simulink library "AEMS_Standard_Library"  (R2016b)
settings: Solver=ode45  StartTime=0.0  StopTime=10.0  RelTol=1e-3
undefined symbols (not defined in the file or in its folder): BkPY, carto, Cbx_extegr, Cbx_lpegrsys, Cbx_portegr, Cnx_bnk_nr_conf, Cnx_cyl_nr_conf, ConfigManagement, configuration_management, Cxx_dcm_io_tmr_end_xxxx, Cxx_dcm_rt_tmr_end, Cxx_DID_xxxx_IO_max, Cxx_DID_xxxx_IO_min, Cxx_egrhsofs, Cxx_vmaniegi, DEM_DEBOUNCE_FREEZE, DEM_DTR_CTL_INVISIBLE, DEM_DTR_CTL_NORMAL, Dem_DtrId2_XXX, Dem_DtrId3_XXX, Dem_DtrId4_XXX, Dem_DtrId5_XXX, Dem_DtrId6_XXX, Dem_DtrId7_XXX, Dem_DtrId8_XXX, Dem_DtrId9_XXX, Dem_DtrId_XXX, Dem_EnableConditionId2_XXX, Dem_EnableConditionId3_XXX, Dem_EnableConditionId4_XXX, Dem_EnableConditionId5_XXX, Dem_EnableConditionId6_XXX, Dem_EnableConditionId7_XXX, Dem_EnableConditionId8_XXX, Dem_EnableConditionId_XXX, Dem_EventId, Dem_EventId2_XXX, Dem_EventId3_XXX, Dem_EventId4_XXX, Dem_EventId5_XXX, Dem_EventId6_XXX, Dem_EventId7_XXX, Dem_EventId8_XXX, Dem_EventId9_XXX, Dem_EventId_Device_Faulttype, Dem_EventId_XXX, DEM_IUMPR_GENERAL_DENOMINATOR, DEM_OPCYC_IGNITION, Dem_RatioId2_XXX, Dem_RatioId3_XXX, Dem_RatioId4_XXX, Dem_RatioId5_XXX, Dem_RatioId6_XXX, Dem_RatioId7_XXX, Dem_RatioId8_XXX, Dem_RatioId_XXX, Dem_StorageConditionId2_XXX, Dem_StorageConditionId3_XXX, Dem_StorageConditionId4_XXX, Dem_StorageConditionId5_XXX ... (+65)
libraries: AEMS_Standard_Library x477, simulink x2
(part 26 of 39)

== system AEMS_Standard_Library/COM/AEMS_FRAME_SUPERVISION/ecu_frm_detection ==
  Clear_Diag_Info : Inport
  Frm_Detection_Cnd : Inport  Port=2
  Frm_Conf : Inport  Port=3
  Status_Loc2 : Inport  Port=4
  AEMS_NVM_SET : AEMS_Standard_Library/MEM/AEMS_NVM_SET  Tag=[LIB]  initial_value=0
      settings: AttributesFormatString=<initial=%<initial_value>>
  C_mngt : Subsystem
      settings: RTWSystemCode=Nonreusable function
  Frame_Detected : Outport
  wires:
  AEMS_NVM_SET/1 -> C_mngt/5(Frm_Detected_PREV)
  C_mngt/1(Frm_Detected) -> AEMS_NVM_SET/1, Frame_Detected/1
  Frm_Detection_Cnd/1 -> C_mngt/1(Frm_Detection_Cnd)
  Frm_Conf/1 -> C_mngt/3(Frm_Conf)
  Status_Loc2/1 -> C_mngt/2(Status_Loc2)
  Clear_Diag_Info/1 -> C_mngt/4(Clear_Diag_Info_Counter)

== system AEMS_Standard_Library/COM/AEMS_FRAME_SUPERVISION/ecu_frm_monitoring ==
  rcpt_frm : Inport
  JT1 : Inport  Port=2
  JT2 : Inport  Port=3
  TimeSched_dt : Inport  Port=4
  GADE : Inport  Port=5
  ECU_Category : Inport  Port=6
  IgnitionSupplyConfirmation : Inport  Port=7
  Specific_Mon_Cnd : Inport  Port=8
  Frame_Detected : Inport  Port=9
  BCM_Status : Inport  Port=10
  USM_Status : Inport  Port=11
  Vbx_atsr_sys_ecu_ini_task10ms : Inport  Port=12
  A_Monitoring_Condition : Subsystem
      settings: RTWSystemCode=Nonreusable function
  B_Status_Management : Subsystem
  Status : Outport
      settings: AttributesFormatString=%<SignalName>
  Mon_Authorize : Outport  Port=2
  wires:
  Vbx_atsr_sys_ecu_ini_task10ms/1 -> B_Status_Management/6(Vbx_atsr_sys_ecu_ini_task10ms)
  rcpt_frm/1 -> B_Status_Management/1(rcpt_frm)
  TimeSched_dt/1 -> B_Status_Management/3(TimeSched_dt)
  JT1/1 -> B_Status_Management/4(JT1)
  JT2/1 -> B_Status_Management/5(JT2)
  Frame_Detected/1 -> A_Monitoring_Condition/5(Frame_Detected_Loc2), B_Status_Management/7(Frame_Detected)
  ECU_Category/1 -> A_Monitoring_Condition/2(ECU_Category)
  Specific_Mon_Cnd/1 -> A_Monitoring_Condition/4(Specific_Mon_Cnd)
  USM_Status/1 -> A_Monitoring_Condition/7(USM_Status)
  IgnitionSupplyConfirmation/1 -> A_Monitoring_Condition/3(IgnitionSupplyConfirmation)
  GADE/1 -> A_Monitoring_Condition/1(GADE)
  BCM_Status/1 -> A_Monitoring_Condition/6(BCM_Status)
  A_Monitoring_Condition/1(Mon_Authorize) -> B_Status_Management/2(Mon_Authorize), Mon_Authorize/1
  B_Status_Management/1(Status) -> Status/1

== system AEMS_Standard_Library/COM/AEMS_FRAME_SUPERVISION/ecu_monitoring_display ==
  rcpt_frm_dspl : Inport
  ClearDiagInfo_dspl : Inport  Port=2
  IGN_Status : Inport  Port=3
  Dspl_Mask_Cnd : Inport  Port=4
  Status : Inport  Port=5
  M_Absent_ini : Inport  Port=6
  decM : Inport  Port=7
  decThres : Inport  Port=8
  VALMAX : Inport  Port=9
  Mon_Authorized : Inport  Port=10
  Vbx_atsr_sys_ecu_ini_task10ms : Inport  Port=11
  Constant2 : Constant  Value=0  OutDataTypeStr=Inherit: Inherit via back propagation
  Constant3 : Constant  Value=false
  D_ctr_mem_max : Subsystem
  E_diag_display : Subsystem
  Switch : Switch  Criteria=u2 ~= 0
      settings: AttributesFormatString=Criteria=%<Criteria>
  Switch1 : Switch  Criteria=u2 ~= 0
      settings: AttributesFormatString=Criteria=%<Criteria>
  Switch2 : Switch  Criteria=u2 ~= 0
      settings: AttributesFormatString=Criteria=%<Criteria>
  Unit Delay : UnitDelay  SampleTime=-1
      settings: AttributesFormatString=<initial=%<InitialCondition>>
  Unit Delay1 : UnitDelay  SampleTime=-1
      settings: AttributesFormatString=<initial=%<InitialCondition>>
  Diagnosis_Byte : Outport
  M_Absent : Outport  Port=2
  wires:
  Unit Delay1/1 -> D_ctr_mem_max/2(M_Absent_PREV)
  Unit Delay/1 -> D_ctr_mem_max/3(Vbx_rcpt_XXX_mon_PREV)
  Switch/1 -> M_Absent/1, E_diag_display/1(M_Absent), Unit Delay1/1
  Switch1/1 -> Unit Delay/1
  ClearDiagInfo_dspl/1 -> D_ctr_mem_max/8(Clear_Diag_Info_Counter)
  rcpt_frm_dspl/1 -> D_ctr_mem_max/7(Frame_Received_Counter)
  Vbx_atsr_sys_ecu_ini_task10ms/1 -> Switch1/2, Switch/2, Switch2/2
  Constant2/1 -> Switch2/1
  E_diag_display/1(Diagnosis_Byte) -> Switch2/3
  Constant3/1 -> Switch1/1
  D_ctr_mem_max/2(Vbx_rcpt_XXX_mon) -> Switch1/3
  M_Absent_ini/1 -> Switch/1
  D_ctr_mem_max/1(M_Absent) -> Switch/3
  Switch2/1 -> Diagnosis_Byte/1
  VALMAX/1 -> D_ctr_mem_max/1(VALMAX)
  Dspl_Mask_Cnd/1 -> E_diag_display/3(Dspl_Mask_Cnd)
  Status/1 -> D_ctr_mem_max/9(Status), E_diag_display/4(Status)
  Mon_Authorized/1 -> E_diag_display/2(Mon_Authorized)
  decM/1 -> D_ctr_mem_max/5(decM)
  decThres/1 -> D_ctr_mem_max/6(decThres)
  IGN_Status/1 -> D_ctr_mem_max/4(IGN_Status)

== system AEMS_Standard_Library/DCM/AEMS_APP_REQUEST_IOCONTROL/Request_IOControl_Subsystem ==
  Req_stadj_xxxx : Inport
  Req_rcecu_xxxx : Inport  Port=2
  Generic_Condition : Inport  Port=3
  Specific_Condition_xxxx : Inport  Port=4
  Req_tmr_end_xxxx : Inport  Port=5
  AEMS_EDGE_RISING : AEMS_Standard_Library/EDGE/AEMS_EDGE_RISING  Tag=[LIB]  init=true
      settings: AttributesFormatString=|
      | %<MaskType>
      | Initial Value : %<init>
  AEMS_SRFLIPFLOP : AEMS_Standard_Library/FLAG/AEMS_SRFLIPFLOP  Tag=[LIB]  init=false
      settings: AttributesFormatString=%<MaskType>\nInitial condition (state of Q): = %<init>
  Logical Operator : Logic  Operator=OR  Inputs=3  OutDataTypeStr=boolean
  Logical Operator1 : Logic  OutDataTypeStr=boolean
  Logical Operator2 : Logic  Operator=NOT  OutDataTypeStr=boolean
  Logical_Operator1 : Logic  Operator=XOR  OutDataTypeStr=boolean
  Logical_Operator4 : Logic  Operator=XOR  OutDataTypeStr=boolean
  Unit Delay : UnitDelay  InitialCondition=false  SampleTime=-1
      settings: AttributesFormatString=<initial=%<InitialCondition>>
  Unit Delay1 : UnitDelay  InitialCondition=false  SampleTime=-1
      settings: AttributesFormatString=<initial=%<InitialCondition>>
  Flag_io_request_xxxx : Outport
  Flag_dcm_io_tmr_end_xxxx : Outport  Port=2
  wires:
  Req_stadj_xxxx/1 -> Logical_Operator4/1, Unit Delay/1
  Unit Delay/1 -> Logical_Operator4/2
  Logical_Operator4/1 -> AEMS_SRFLIPFLOP/1
  Req_rcecu_xxxx/1 -> Logical_Operator1/1, Unit Delay1/1
  Generic_Condition/1 -> Logical Operator1/1
  Specific_Condition_xxxx/1 -> Logical Operator1/2
  Unit Delay1/1 -> Logical_Operator1/2
  Logical_Operator1/1 -> Logical Operator/1
  Logical Operator/1 -> AEMS_SRFLIPFLOP/2
  Logical Operator1/1 -> Logical Operator2/1
  Logical Operator2/1 -> Logical Operator/2
  AEMS_SRFLIPFLOP/1 -> Flag_io_request_xxxx/1
  Req_tmr_end_xxxx/1 -> AEMS_EDGE_RISING/1
  AEMS_EDGE_RISING/1 -> Logical Operator/3, Flag_dcm_io_tmr_end_xxxx/1

== system AEMS_Standard_Library/DCM/AEMS_APP_REQUEST_IOCONTROL/Timer_IOControl_Subsystem ==
  note: Reset Threshold value defined in
      | Cxx_dcm_io_tmr_end_xxxx whenever
      | a edge raising or failing detected
  note: Decrementation:
      | Decrement 10 milisecondes from Calibration High_Threshold to 0 and set the Duration of Timer
      | Decrement every 10MS
  note: Set Timer value
      | Set Timer_End if Duration reached
  Req_stadj_xxxx : Inport
  Constant : Constant  Value=0  OutDataTypeStr=single
  Cxx_dcm_io_tmr_end_xxxx : Constant  Value=Cxx_dcm_io_tmr_end_xxxx  OutDataTypeStr=single
  Increment : Constant  Value=10  OutDataTypeStr=single
  Logical_Operator4 : Logic  Operator=XOR  OutDataTypeStr=boolean
  MinMax : MinMax  Function=max  Inputs=2
  Relational Operator : RelationalOperator  Operator=<=  OutDataTypeStr=boolean  RndMeth=Nearest  InputSameDT=on
  Saturation : Saturate  UpperLimit=655350  LowerLimit=0
      settings: AttributesFormatString=<limits=%<UpperLimit>/%<LowerLimit>>
  Sum : Sum  Inputs=-+  OutDataTypeStr=single  SaturateOnIntegerOverflow=on  InputSameDT=on
      settings: AttributesFormatString=SAT = %<SaturateOnIntegerOverflow>
  Switch : Switch  Criteria=u2 ~= 0
      settings: AttributesFormatString=Criteria=%<Criteria>
  Unit Delay : UnitDelay  InitialCondition=false  SampleTime=-1
      settings: AttributesFormatString=<initial=%<InitialCondition>>
  Unit Delay1 : UnitDelay  SampleTime=-1
      settings: AttributesFormatString=<initial=%<InitialCondition>>
  Req_tmr_end_xxxx : Outport
  Dcm_io_tmr_xxxx : Outport  Port=2
  wires:
  Req_stadj_xxxx/1 -> Logical_Operator4/1, Unit Delay/1
  Unit Delay/1 -> Logical_Operator4/2
  Constant/1 -> Relational Operator/2
  Increment/1 -> MinMax/1, Sum/1
  Switch/1 -> Saturation/1
  Sum/1 -> Switch/3
  Logical_Operator4/1 -> Switch/2
  Unit Delay1/1 -> MinMax/2
  MinMax/1 -> Sum/2
  Relational Operator/1 -> Req_tmr_end_xxxx/1
  Cxx_dcm_io_tmr_end_xxxx/1 -> Switch/1
  Saturation/1 -> Unit Delay1/1, Relational Operator/1, Dcm_io_tmr_xxxx/1

== system AEMS_Standard_Library/DCM/AEMS_APP_REQUEST_IOCONTROL/Write_IOControl_Subsystem ==
  Value_Write_stadj_xxxx : Inport
  Data Type Conversion : DataTypeConversion
  Val_io_request_xxxx : Outport
  wires:
  Value_Write_stadj_xxxx/1 -> Data Type Conversion/1
  Data Type Conversion/1 -> Val_io_request_xxxx/1

== system AEMS_Standard_Library/DCM/AEMS_APP_REQUEST_ROUTINE/Request_Routine_Subsystem ==
  Req_sta_xxxx : Inport
  Req_stop_xxxx : Inport  Port=2
  Generic_Condition : Inport  Port=3
  Specific_Condition_xxxx : Inport  Port=4
  Flag_req_tmr_end : Inport  Port=5
  AEMS_EDGE_RISING : AEMS_Standard_Library/EDGE/AEMS_EDGE_RISING  Tag=[LIB]  init=false
      settings: AttributesFormatString=|
      | %<MaskType>
      | Initial Value : %<init>
  Logical Operator4 : Logic  OutDataTypeStr=boolean
  Logical Operator5 : Logic  Operator=OR  OutDataTypeStr=boolean
  Logical Operator6 : Logic  Operator=NOT  OutDataTypeStr=boolean
  Logical_Operator1 : Logic  Operator=XOR  OutDataTypeStr=boolean
  Logical_Operator4 : Logic  Operator=XOR  OutDataTypeStr=boolean
  Unit Delay : UnitDelay  SampleTime=-1
      settings: AttributesFormatString=<initial=%<InitialCondition>>
  Unit Delay1 : UnitDelay  SampleTime=-1
      settings: AttributesFormatString=<initial=%<InitialCondition>>
  Flag_sta_xxxx : Outport
  Flag_stop_xxxx : Outport  Port=2
  Flag_dcm_rt_tmr_end : Outport  Port=3
  wires:
  AEMS_EDGE_RISING/1 -> Flag_dcm_rt_tmr_end/1
  Flag_req_tmr_end/1 -> AEMS_EDGE_RISING/1
  Unit Delay/1 -> Logical_Operator4/2
  Logical_Operator4/1 -> Flag_sta_xxxx/1
  Req_stop_xxxx/1 -> Unit Delay1/1, Logical_Operator1/1
  Unit Delay1/1 -> Logical_Operator1/2
  Generic_Condition/1 -> Logical Operator4/1
  Specific_Condition_xxxx/1 -> Logical Operator4/2
  Logical Operator4/1 -> Logical Operator6/1
  Logical Operator6/1 -> Logical Operator5/2
  Logical Operator5/1 -> Flag_stop_xxxx/1
  Logical_Operator1/1 -> Logical Operator5/1
  Req_sta_xxxx/1 -> Unit Delay/1, Logical_Operator4/1

== system AEMS_Standard_Library/DCM/AEMS_APP_REQUEST_ROUTINE/Timer_routine_Subsystem ==
  note: Set Timer value by converting from 10MS to 100MS
      | Set Timer_End if Duration reached
  note: Decrementation:
      | Convert Calibration Cxx from unit 100MS to 10MS and set the Duration of Timer
      | Decrement every 10MS
  note: Activation of decrementation whenever
      | a edge raising or failing detected
  Req_sta_xxxx : Inport
  Constant : Constant  Value=0  OutDataTypeStr=single
  Constant1 : Constant  Value=100  OutDataTypeStr=single
  Constant2 : Constant  OutDataTypeStr=single
  Cxx_dcm_rt_tmr_end : Constant  Value=Cxx_dcm_rt_tmr_end  OutDataTypeStr=single
  Divide : Product  Inputs=*/  OutDataTypeStr=single
  Factor1 : Constant  Value=100  OutDataTypeStr=single
  Logical_Operator4 : Logic  Operator=XOR  OutDataTypeStr=boolean
  MinMax : MinMax  Function=max  Inputs=2
  Product : Product  OutDataTypeStr=single
  Relational Operator : RelationalOperator  Operator===  OutDataTypeStr=boolean  RndMeth=Nearest  InputSameDT=on
  Saturation : Saturate  UpperLimit=655350  LowerLimit=0
      settings: AttributesFormatString=<limits=%<UpperLimit>/%<LowerLimit>>
  Sum : Sum  Inputs=-+  OutDataTypeStr=single  InputSameDT=on
  Switch : Switch  Criteria=u2 ~= 0
      settings: AttributesFormatString=Criteria=%<Criteria>
  Unit Delay : UnitDelay  SampleTime=-1
      settings: AttributesFormatString=<initial=%<InitialCondition>>
  Unit Delay1 : UnitDelay  SampleTime=-1
      settings: AttributesFormatString=<initial=%<InitialCondition>>
  Flag_req_tmr_end : Outport
  Dcm_rt_tmr : Outport  Port=2
  wires:
  Divide/1 -> Dcm_rt_tmr/1
  Factor1/1 -> Divide/2
  Cxx_dcm_rt_tmr_end/1 -> Product/1
  Constant1/1 -> Product/2
  MinMax/1 -> Sum/2
  Unit Delay1/1 -> MinMax/2
  Logical_Operator4/1 -> Switch/2
  Sum/1 -> Switch/3
  Switch/1 -> Saturation/1
  Constant2/1 -> Sum/1, MinMax/1
  Constant/1 -> Relational Operator/2
  Relational Operator/1 -> Flag_req_tmr_end/1
  Saturation/1 -> Divide/1, Relational Operator/1, Unit Delay1/1
  Product/1 -> Switch/1
  Unit Delay/1 -> Logical_Operator4/2
  Req_sta_xxxx/1 -> Unit Delay/1, Logical_Operator4/1

== system AEMS_Standard_Library/DCM/AEMS_DCM_CLEARDIAGNOSTICINFORMATION/Callback_Subsystem ==
  note: Request
  note: Client / Server
  note: ERRORCode
  note: E_NOT_OK
  note: E_OK
  Condition : Inport
  Constant1 : Constant  Description=NRC22  Value=0  OutDataTypeStr=uint8  SampleTime=-1
  Constant2 : Constant  Description=NRC22  Value=34  OutDataTypeStr=uint8  SampleTime=-1
      settings: AttributesFormatString=%<Description>
  Constant3 : Constant  Value=0  OutDataTypeStr=uint8  SampleTime=-1
  DataTypeConversion : DataTypeConversion  RndMeth=Zero
  Enable_Clear_Request_Subsystem : Subsystem
  Logical Operator3 : Logic  Operator=NOT  OutDataTypeStr=boolean
  NRC1 : Constant  Description=NRC22  OutDataTypeStr=uint8  SampleTime=-1
  Switch : Switch  Criteria=u2 ~= 0
      settings: AttributesFormatString=Criteria=%<Criteria>
  Switch1 : Switch  Criteria=u2 ~= 0
      settings: AttributesFormatString=Criteria=%<Criteria>
  flag_clr_req : Outport
  ErrorCode : Outport  Port=2
  Std_ReturnType : Outport  Port=3
  wires:
  Switch/1 -> ErrorCode/1
  Constant1/1 -> Switch1/1
  NRC1/1 -> Switch1/3
  Switch1/1 -> Std_ReturnType/1  "Std_ReturnType"
  Constant3/1 -> Switch/1
  Constant2/1 -> Switch/3
  Enable_Clear_Request_Subsystem/1(flag_clr_req) -> DataTypeConversion/1
  Condition/1 -> Logical Operator3/1
  Logical Operator3/1 -> Switch1/2, Enable_Clear_Request_Subsystem/Enable, Switch/2
  DataTypeConversion/1 -> flag_clr_req/1

== system AEMS_Standard_Library/DCM/AEMS_DCM_CONDITIONCHECKREAD/Callback_Subsystem ==
  note: NRC22
  note: CLIENT/SERVER:
      |
      | ErrorCode:
      | another routine is already running ErrorCode = 34
      | else ErrorCode = 0
  note: Negative response code computation
  note: E_OK
  note: E_NOT_OK
  Condition_checkread : Inport
  Constant1 : Constant  Description=NRC22  Value=0  OutDataTypeStr=uint8  SampleTime=-1
  Constant2 : Constant  Description=NRC22  Value=0  OutDataTypeStr=uint8  SampleTime=-1
  NRC1 : Constant  Description=NRC22  OutDataTypeStr=uint8  SampleTime=-1
  NRC22 : Constant  Description=NRC22  Value=34  OutDataTypeStr=uint8  SampleTime=-1
  Switch1 : Switch  Criteria=u2 ~= 0
      settings: AttributesFormatString=Criteria=%<Criteria>
  Switch2 : Switch  Criteria=u2 ~= 0
      settings: AttributesFormatString=Criteria=%<Criteria>
  ErrorCode : Outport
  Std_ReturnType : Outport  Port=2
  wires:
  NRC1/1 -> Switch1/3
  Constant1/1 -> Switch1/1
  Switch1/1 -> Std_ReturnType/1  "Std_ReturnType"
  Switch2/1 -> ErrorCode/1  "ErrorCode"
  Condition_checkread/1 -> Switch2/2, Switch1/2
  Constant2/1 -> Switch2/1
  NRC22/1 -> Switch2/3

== system AEMS_Standard_Library/DCM/AEMS_DCM_DID_READDATA/Callback_Subsystem ==
  note: E_OK
  Value_Read_xxxx_DCM : Inport
  Constant1 : Constant  Description=NRC22  Value=0  OutDataTypeStr=uint8  SampleTime=-1
  Data : Outport  OutDataTypeStr=uint8
  Std_ReturnType : Outport  Port=2  OutDataTypeStr=uint8
  wires:
  Constant1/1 -> Std_ReturnType/1  "Std_ReturnType"
  Value_Read_xxxx_DCM/1 -> Data/1  "Data"

== system AEMS_Standard_Library/DCM/AEMS_DCM_DID_READDATA/Conversion_Subsystem ==
  DID_Variable_1 : Inport
  AEMS_EXTRACT_BIT_1 : AEMS_Standard_Library/BIT_OPERATION/AEMS_EXTRACT_BIT  Tag=[LIB]  Description=NOTE: The value of 'Number of bits' must be between 0 to 31.  DataType=uint8  Value=Range of bits  Range=[0,7]  NB=28
      settings: AttributesFormatString="%<MaskType>\\nBits to extract = %<Value>\\nInput data type  = %<DataType>\\nRange of Bit: = %<Range>"
  AEMS_TO_FXP_WITH_LIMIT_1 : AEMS_Standard_Library/DCM/AEMS_TO_FXP_WITH_LIMIT  Tag=[LIB]  Resol=1  Min=0  Max=255  OutputFixedPointDatatype=uint8  Offset=0
      settings: AttributesFormatString=%<MaskType>\nResolution (physical) = %<Resol>\nOffset (Physical) = %<Offset>\nMinimum (Physical) = %<Min>\nMaximum (Physical) = %<Max>\nOutput Fixed Point Datatype=%<OutputFixedPointDatatype>
  Mux : Mux  Inputs=1
  Value_Read_xxxx_DCM : Outport
  wires:
  Mux/1 -> Value_Read_xxxx_DCM/1
  DID_Variable_1/1 -> AEMS_TO_FXP_WITH_LIMIT_1/1
  AEMS_TO_FXP_WITH_LIMIT_1/1 -> AEMS_EXTRACT_BIT_1/1
  AEMS_EXTRACT_BIT_1/1 -> Mux/1

== system AEMS_Standard_Library/DCM/AEMS_DCM_DID_WRITEDATA/Callback_Subsystem ==
  note: E_OK
  note: E_NOT_OK
  note: ERRORCode
  note: Client / Server
  note: Request
  note: case 1 : permission = 1 and previous request = 0 (init = 0)
      | 	x = permission AND NOT(previous request) = 1
      | 	y = NOT(permission) AND previous request = 1
      | 	x OR y = 1 so request = 1
      |
      | case 2 : Permission = 1 and previous request = 1
      | 	x = permission AND NOT(previous request) = 0
      | 	y = NOT(permission) AND previous request = 0
      | 	x OR y = 0 so request = 0
      |
      | case 3 : permission = 0 and previous request = 0
      | 	x = permission AND NOT(previous request) = 0
      | 	y = NOT(permission) AND previous request = 0
      | 	x OR y = 1 so request = 0
      |
      | case 4 : permission = 0 and previous request = 1
      | 	x = permission AND NOT(previous request) = 1
      | 	y = NOT(permission) AND previous request = 1
      | 	x OR y = 1 so request = 1
  Permission : Inport
  "ConfigMgmt " : Constant  Value=ConfigManagement  OutDataTypeStr=boolean
  Constant1 : Constant  Description=NRC22  Value=0  OutDataTypeStr=uint8
  Constant2 : Constant  Description=NRC22  Value=34  OutDataTypeStr=uint8
      settings: AttributesFormatString=%<Description>
  Constant3 : Constant  Value=0  OutDataTypeStr=uint8
  Logical Operator : Logic  OutDataTypeStr=boolean
  Logical Operator1 : Logic  Operator=OR  OutDataTypeStr=boolean
  Logical Operator2 : Logic  Operator=NOT  OutDataTypeStr=boolean
  Logical Operator3 : Logic  Operator=NOT  OutDataTypeStr=boolean
  Logical Operator4 : Logic  OutDataTypeStr=boolean
  Logical Operator5 : Logic  OutDataTypeStr=boolean
  NRC1 : Constant  Description=NRC22  OutDataTypeStr=uint8
  Switch : Switch  Criteria=u2 ~= 0
      settings: AttributesFormatString=Criteria=%<Criteria>
  Switch1 : Switch  Criteria=u2 ~= 0
      settings: AttributesFormatString=Criteria=%<Criteria>
  Unit Delay1 : UnitDelay  SampleTime=-1
      settings: AttributesFormatString=<initial=%<InitialCondition>>
  Request_Write_xxxx_DCM : Outport
  ErrorCode : Outport  Port=2
  Std_ReturnType : Outport  Port=3
  wires:
  NRC1/1 -> Switch1/3
  Constant1/1 -> Switch1/1
  Switch1/1 -> Std_ReturnType/1  "Std_ReturnType"
  Logical Operator5/1 -> Logical Operator2/1, Logical Operator/1, Switch/2, Switch1/2
  Unit Delay1/1 -> Logical Operator4/2, Logical Operator3/1
  Logical Operator2/1 -> Logical Operator4/1
  Logical Operator3/1 -> Logical Operator/2
  Logical Operator1/1 -> Request_Write_xxxx_DCM/1, Unit Delay1/1
  Logical Operator/1 -> Logical Operator1/1
  Logical Operator4/1 -> Logical Operator1/2
  Constant2/1 -> Switch/3
  Constant3/1 -> Switch/1
  "ConfigMgmt "/1 -> Logical Operator5/2
  Permission/1 -> Logical Operator5/1
  Switch/1 -> ErrorCode/1

== system AEMS_Standard_Library/DCM/AEMS_DCM_DID_WRITEDATA/Permission_Subsystem ==
  Generic_conditions_Write : Inport
  Specific_conditions_Write_xxxx : Inport  Port=2
  Logical Operator : Logic  OutDataTypeStr=boolean
  Permission : Outport
  wires:
  Generic_conditions_Write/1 -> Logical Operator/1
  Specific_conditions_Write_xxxx/1 -> Logical Operator/2
  Logical Operator/1 -> Permission/1

== system AEMS_Standard_Library/DCM/AEMS_DCM_GETPROGCONDITIONS/Callback_Subsystem ==
  note: CLIENT/SERVER:
      |
      | In structure ProgConditions:
      | Only ReprogramingRequest is updated by input Flag_request
      | Remainding element of structure ProgConditions will not be changed.
  note: DCM_COLD_START
  note: Client / Server
  note: Structure of ProgConditions
  Flag_request : Inport
  Bus Creator : BusCreator  Inputs=7
  ConnectionId{,1..3,5..6} (6 alike) : Ground
  Constant1 : Constant  Description=NRC22  Value=0  OutDataTypeStr=uint8  SampleTime=-1
  Data Type Conversion : DataTypeConversion
  ProgConditions : Outport
  Dcm_EcuStartModeType : Outport  Port=2
  wires:
  Data Type Conversion/1 -> Bus Creator/5  "ReprogramingRequest"
  ConnectionId2/1 -> Bus Creator/3  "Sid"
  ConnectionId3/1 -> Bus Creator/4  "SubFncId"
  Flag_request/1 -> Data Type Conversion/1
  ConnectionId5/1 -> Bus Creator/6  "ApplUpdated"
  ConnectionId6/1 -> Bus Creator/7  "ResponseRequired"
  ConnectionId1/1 -> Bus Creator/2  "TesterAddress"
  ConnectionId/1 -> Bus Creator/1  "ConnectionId"
  Bus Creator/1 -> ProgConditions/1
  Constant1/1 -> Dcm_EcuStartModeType/1  "Dcm_EcuStartModeType"

== system AEMS_Standard_Library/DCM/AEMS_DCM_GETSESCTRLTYPE/Callback_Subsystem ==
  note: E_OK
  SesCtrlType : Inport
  Constant1 : Constant  Description=NRC22  Value=0  OutDataTypeStr=uint8  SampleTime=-1
  Data : Outport  OutDataTypeStr=uint8
  Std_ReturnType : Outport  Port=2  OutDataTypeStr=uint8
  wires:
  SesCtrlType/1 -> Data/1  "Data"
  Constant1/1 -> Std_ReturnType/1  "Std_ReturnType"

== system AEMS_Standard_Library/DCM/AEMS_DCM_IO_RETURN_CONTROL_TO_ECU/Callback_Subsystem ==
  note: E_OK
  note: Request
  Constant : Constant  Value=0  OutDataTypeStr=uint8
  Constant1 : Constant  Description=NRC22  Value=0  OutDataTypeStr=uint8  SampleTime=-1
  ErrorCode : Outport
  Std_ReturnType : Outport  Port=2
  wires:
  Constant1/1 -> Std_ReturnType/1  "Std_ReturnType"
  Constant/1 -> ErrorCode/1  "ErrorCode"

== system AEMS_Standard_Library/DCM/AEMS_DCM_IO_SHORT_TERM_ADJUSTMENT/Callback_Subsystem ==
  note: CONDITION:
      |
      | case 1 : permission = 1 and previous request = 0 (init = 0)
      | 	x = permission AND NOT(previous request) = 1
      | 	y = NOT(permission) AND previous request = 1
      | 	x OR y = 1 so request = 1
      |
      | case 2 : Permission = 1 and previous request = 1
      | 	x = permission AND NOT(previous request) = 0
      | 	y = NOT(permission) AND previous request = 0
      | 	x OR y = 0 so request = 0
      |
      | case 3 : permission = 0 and previous request = 0
      | 	x = permission AND NOT(previous request) = 0
      | 	y = NOT(permission) AND previous request = 0
      | 	x OR y = 1 so request = 0
      |
      | case 4 : permission = 0 and previous request = 1
      | 	x = permission AND NOT(previous request) = 1
      | 	y = NOT(permission) AND previous request = 1
      | 	x OR y = 1 so request = 1
  note: Negative response code computation
  note: Client / Server
  note: Request
  note: DID Write in FLP
  note: XOR
  note: E_NOT_OK
  note: E_OK
  Permission : Inport
  ControlStateInfo_flp : Inport  Port=2
  Configuration_management : Constant  Value=configuration_management  OutDataTypeStr=boolean
  "Const " : Constant  Value=0  OutDataTypeStr=uint8
  Const 1 : Constant  Value=0  OutDataTypeStr=uint8
  Const2 : Constant  Value=0  OutDataTypeStr=uint8
  Constant1 : Constant  Description=NRC22  Value=0  OutDataTypeStr=uint8
  Constant2 : Constant  Description=NRC22  Value=34  OutDataTypeStr=uint8
      settings: AttributesFormatString=%<Description>
  Cxx_DID_xxxx_IO_max : Constant  Value=Cxx_DID_xxxx_IO_max  OutDataTypeStr=Inherit: Inherit via back propagation
  Cxx_DID_xxxx_IO_min : Constant  Value=Cxx_DID_xxxx_IO_min  OutDataTypeStr=Inherit: Inherit via back propagation
  Logical Operator{,4..6} (4 alike) : Logic  OutDataTypeStr=boolean
  Logical Operator1 : Logic  Operator=OR  OutDataTypeStr=boolean
  Logical Operator2 : Logic  Operator=NOT  OutDataTypeStr=boolean
  Logical Operator3 : Logic  Operator=NOT  OutDataTypeStr=boolean
  NRC1 : Constant  Description=NRC22  OutDataTypeStr=uint8
  NRC31 : Constant  Value=49  OutDataTypeStr=uint8
      settings: AttributesFormatString=%<Name>
  Relational Operator1 : RelationalOperator  Operator=<  OutDataTypeStr=boolean  RndMeth=Nearest  InputSameDT=on
  Relational Operator2 : RelationalOperator  Operator=>  OutDataTypeStr=boolean  RndMeth=Nearest  InputSameDT=on
  Relational Operator3 : RelationalOperator  Operator===  OutDataTypeStr=boolean  RndMeth=Nearest  InputSameDT=on
  Relational Operator4 : RelationalOperator  Operator=>  OutDataTypeStr=boolean  RndMeth=Nearest  InputSameDT=on
  Switch{,1..3} (4 alike) : Switch  Criteria=u2 ~= 0
      settings: AttributesFormatString=Criteria=%<Criteria>
  Unit Delay1 : UnitDelay  SampleTime=-1
      settings: AttributesFormatString=<initial=%<InitialCondition>>
  Value_Write_xxxx_DCM : Outport
  ShortTermAdjustement_flag_Request_xxxx_DCM : Outport  Port=2
  ErrorCode : Outport  Port=3
  Std_ReturnType : Outport  Port=4
  wires:
  Logical Operator6/1 -> Logical Operator/1, Logical Operator2/1
  Relational Operator3/1 -> Logical Operator6/2
  ControlStateInfo_flp/1 -> Relational Operator1/1, Relational Operator2/1, Value_Write_xxxx_DCM/1
  Cxx_DID_xxxx_IO_max/1 -> Relational Operator2/2
  Logical Operator5/1 -> Switch/2, Logical Operator6/1
  Switch/1 -> Relational Operator4/1, ErrorCode/1  "ErrorCode"
  Switch2/1 -> Switch/1, Relational Operator3/2
  Constant2/1 -> Switch/3
  Const2/1 -> Relational Operator3/1
  Switch1/1 -> Switch2/3
  Relational Operator1/1 -> Switch2/2
  Cxx_DID_xxxx_IO_min/1 -> Relational Operator1/2
  "Const "/1 -> Switch1/3
  NRC31/1 -> Switch2/1, Switch1/1
  Relational Operator2/1 -> Switch1/2
  Permission/1 -> Logical Operator5/1
  Configuration_management/1 -> Logical Operator5/2
  Logical Operator4/1 -> Logical Operator1/2
  Logical Operator/1 -> Logical Operator1/1
  Logical Operator3/1 -> Logical Operator/2
  Logical Operator2/1 -> Logical Operator4/1
  Unit Delay1/1 -> Logical Operator3/1, Logical Operator4/2
  Logical Operator1/1 -> ShortTermAdjustement_flag_Request_xxxx_DCM/1, Unit Delay1/1
  Relational Operator4/1 -> Switch3/2
  Switch3/1 -> Std_ReturnType/1  "Std_ReturnType"
  Constant1/1 -> Switch3/3
  NRC1/1 -> Switch3/1
  Const 1/1 -> Relational Operator4/2

== system AEMS_Standard_Library/DCM/AEMS_DCM_IO_SHORT_TERM_ADJUSTMENT/Conversion_Subsystem ==
  note: Conversion from buffer in uint8 to scalar in FXP:
      |
      | ControlStateInfo written by DCM in array form and converted to
      | a scalar in FXP by multiplied by factor [1 2^8 2^16 2^24] depend on size of DID
  note: ControlStateInfo in buffer
  note: Value_FLP
  ControlStateInfo : Inport
  Conversion_Subsystem : AEMS_Standard_Library/SUB/AEMS_CONVERT_BYTE_TO_FLP  Tag=[LIB]  Resol=1  offset=0  DID_Datatype=uint8
      settings: AttributesFormatString=%<MaskType>\nResolution = %<Resol>\nOffset = %<offset>\nDIDType = %<DID_DataType>
  Data Type Conversion1 : DataTypeConversion  OutDataTypeStr=uint8  RndMeth=Zero
  Demux : Demux  Outputs=[1]
  ControlStateInfo_flp : Outport
  wires:
  ControlStateInfo/1 -> Data Type Conversion1/1
  Conversion_Subsystem/1 -> ControlStateInfo_flp/1
  Demux/1 -> Conversion_Subsystem/1
  Data Type Conversion1/1 -> Demux/1

== system AEMS_Standard_Library/DCM/AEMS_DCM_IO_SHORT_TERM_ADJUSTMENT/Permission_Subsystem ==
  Generic_Conditions_RoutineIO : Inport
  Specific_Conditions_IO_XXXX : Inport  Port=2
  Logical Operator : Logic  OutDataTypeStr=boolean
  Permission : Outport
  wires:
  Logical Operator/1 -> Permission/1
  Specific_Conditions_IO_XXXX/1 -> Logical Operator/2
  Generic_Conditions_RoutineIO/1 -> Logical Operator/1

== system AEMS_Standard_Library/DCM/AEMS_DCM_REQUEST_RESULT/Callback_Subsystem ==
  note: CLIENT/SERVER:
      |
      | ErrorCode:
      | ErrorCode = 0
      |
      |
      | Routine STOP Control Response:
      | Routine Status = 1 (disabled), 2 (running), 0 (completed)
      | Routine Type = 3 for Renault
      | Two these values are stored in one byte dataOut_1 in which 4 LSB are for
      | Routine Status and 4 MSB are for Routine Type
      | Example: Routine Status = 1 (disabled)
      | Routine Type = 3 for Renault
      | dataOut_1: Routine Status + 2^4*Routine Type (2^4 shift 4 bits)
      | dataOut_1: 1+3*16=49
  note: E_OK
  Routine_xxxx_Status : Inport
  Add : Sum  OutDataTypeStr=uint8  InputSameDT=on
  Constant1 : Constant  Description=NRC22  Value=0  OutDataTypeStr=uint8
  Constant2 : Constant  Value=Routine_Type_xxxx
  Product : Product  OutDataTypeStr=Inherit: Inherit via back propagation
  Shift3bits : Constant  Value=16  OutDataTypeStr=uint8
  Shift3bits1 : Constant  Value=0  OutDataTypeStr=uint8
  dataOut_1 : Outport
  ErrorCode : Outport  Port=2
  Std_ReturnType : Outport  Port=3
  wires:
  Constant2/1 -> Product/1
  Shift3bits/1 -> Product/2
  Product/1 -> Add/2
  Add/1 -> dataOut_1/1
  Routine_xxxx_Status/1 -> Add/1
  Shift3bits1/1 -> ErrorCode/1  "ErrorCode"
  Constant1/1 -> Std_ReturnType/1

== system AEMS_Standard_Library/DCM/AEMS_DCM_START_ROUTINE/Callback_Subsystem ==
  note: Do nothing for argument OpStatus
  note: Negative response code computation
  note: case 1 : permission = 1 and previous request = 0 (init = 0)
      | 	x = permission AND NOT(previous request) = 1
      | 	y = NOT(permission) AND previous request = 1
      | 	x OR y = 1 so request = 1
      |
      | case 2 : Permission = 1 and previous request = 1
      | 	x = permission AND NOT(previous request) = 0
      | 	y = NOT(permission) AND previous request = 0
      | 	x OR y = 0 so request = 0
      |
      | case 3 : permission = 0 and previous request = 0
      | 	x = permission AND NOT(previous request) = 0
      | 	y = NOT(permission) AND previous request = 0
      | 	x OR y = 1 so request = 0
      |
      | case 4 : permission = 0 and previous request = 1
      | 	x = permission AND NOT(previous request) = 1
      | 	y = NOT(permission) AND previous request = 1
      | 	x OR y = 1 so request = 1
  note: CLIENT/SERVER:
      |
      | ErrorCode:
      | another routine is already running ErrorCode = 34
      | same routine is already running ErrorCode = 36
      | else ErrorCode = 0
      |
      |
      | Routine STOP Control Response:
      | Routine Status = 0 (disabled), 1(aborted), 2 (running), 3 completed
      | Routine Type = 3 for Renault
      | Two these values are stored in one byte dataOut_1 in which 4 LSB are for
      | Routine Status and 4 MSB are for Routine Type
      | Example: Routine Status = 1 (disabled)
      | Routine Type = 3 for Renault
      | dataOut_1: Routine Status + 2^4*Routine Type (2^4 shift 4 bits)
      | dataOut_1: 1+3*16=49
  note: NRC22
  note: NRC24
  note: NRC24
  note: NRC22
  note: E_NOT_OK
  note: E_OK
  Permission : Inport
  Routine_Status : Inport  Port=2
  Routine_xxxx_Status : Inport  Port=3
  OpStatus : Inport  Port=4
  Add : Sum  OutDataTypeStr=uint8  SaturateOnIntegerOverflow=on  InputSameDT=on
      settings: AttributesFormatString=SAT = %<SaturateOnIntegerOverflow>
  Constant1 : Constant  Description=NRC22  Value=0  OutDataTypeStr=uint8
  Constant2 : Constant  Description=NRC22  Value=0  OutDataTypeStr=uint8
  Constant6 : Constant  Value=Routine_Type_xxxx
  ErrorCode1 : Terminator
  Logical Operator : Logic  OutDataTypeStr=boolean
  Logical Operator1 : Logic  Operator=OR  OutDataTypeStr=boolean
  Logical Operator{2..3,6,8} (4 alike) : Logic  Operator=NOT  OutDataTypeStr=boolean
  Logical Operator4 : Logic  OutDataTypeStr=boolean
  Logical Operator5 : Logic  Operator=OR  OutDataTypeStr=boolean
  Logical Operator7 : Logic  OutDataTypeStr=boolean
  NRC1 : Constant  Description=NRC22  OutDataTypeStr=uint8
  NRC22 : Constant  Description=NRC22  Value=34  OutDataTypeStr=uint8
  NRC22_01 : Constant  Value=34  OutDataTypeStr=uint8
  NRC24 : Constant  Value=36  OutDataTypeStr=uint8
  NRC24_01 : Constant  Value=36  OutDataTypeStr=uint8
  Product : Product  OutDataTypeStr=Inherit: Inherit via back propagation  SaturateOnIntegerOverflow=on
      settings: AttributesFormatString=SAT = %<SaturateOnIntegerOverflow>
  Relational Operator1 : RelationalOperator  Operator===  OutDataTypeStr=boolean  RndMeth=Nearest  InputSameDT=on
  Relational Operator2 : RelationalOperator  Operator===  OutDataTypeStr=boolean  RndMeth=Nearest  InputSameDT=on
  Relational Operator3 : RelationalOperator  Operator===  OutDataTypeStr=boolean  RndMeth=Nearest  InputSameDT=on
  Routine_xxxx_Status_Running : Constant  Value=Routine_Status_Running
  Routine_xxxx_Status_disable : Constant  Value=Routine_Status_Aborted
  Shift3bits : Constant  Value=16  OutDataTypeStr=uint8
  Switch{1..4} (4 alike) : Switch  Criteria=u2 ~= 0
      settings: AttributesFormatString=Criteria=%<Criteria>
  Unit Delay1 : UnitDelay  SampleTime=-1
      settings: AttributesFormatString=<initial=%<InitialCondition>>
  Flag_request_xxxx_DCM : Outport
  dataOut_1 : Outport  Port=2
  ErrorCode : Outport  Port=3
  Std_ReturnType : Outport  Port=4
  wires:
  Logical Operator1/1 -> Flag_request_xxxx_DCM/1, Unit Delay1/1
  Unit Delay1/1 -> Logical Operator4/2, Logical Operator3/1
  Logical Operator2/1 -> Logical Operator4/1
  Logical Operator3/1 -> Logical Operator/2
  Logical Operator/1 -> Logical Operator1/1
  Logical Operator4/1 -> Logical Operator1/2
  Permission/1 -> Logical Operator2/1, Logical Operator/1, Logical Operator7/1
  Routine_xxxx_Status/1 -> Relational Operator1/1
  Switch2/1 -> Switch1/1
  NRC22/1 -> Switch2/3
  Constant2/1 -> Switch2/1
  Logical Operator8/1 -> Switch1/2
  Relational Operator1/1 -> Logical Operator8/1
  NRC24/1 -> Switch1/3
  Logical Operator6/1 -> Logical Operator7/2
  Logical Operator7/1 -> Switch2/2
  Switch1/1 -> ErrorCode/1, Relational Operator2/2, Relational Operator3/1  "ErrorCode"
  Switch4/1 -> Add/1
  Routine_xxxx_Status_disable/1 -> Switch4/1
  NRC24_01/1 -> Relational Operator2/1
  Routine_xxxx_Status_Running/1 -> Relational Operator1/2, Switch4/3
  Routine_Status/1 -> Logical Operator6/1
  NRC22_01/1 -> Relational Operator3/2
  Relational Operator2/1 -> Logical Operator5/1
  Relational Operator3/1 -> Logical Operator5/2
  Shift3bits/1 -> Product/2
  Product/1 -> Add/2
  Add/1 -> dataOut_1/1  "dataOut_1"
  Constant6/1 -> Product/1
  OpStatus/1 -> ErrorCode1/1
  Logical Operator5/1 -> Switch3/2, Switch4/2
  Switch3/1 -> Std_ReturnType/1  "Std_ReturnType"
  NRC1/1 -> Switch3/1
  Constant1/1 -> Switch3/3

== system AEMS_Standard_Library/DCM/AEMS_DCM_START_ROUTINE/Permission_Subsystem ==
  Generic_Conditions_Routine : Inport
  Specific_Conditions_Routine_xxxx : Inport  Port=2
  Routine_Status : Inport  Port=3
  Logical Operator : Logic  Inputs=3  OutDataTypeStr=boolean
  Logical Operator6 : Logic  Operator=NOT  OutDataTypeStr=boolean
  Permission : Outport
  wires:
  Generic_Conditions_Routine/1 -> Logical Operator/1
  Specific_Conditions_Routine_xxxx/1 -> Logical Operator/2
  Logical Operator/1 -> Permission/1
  Logical Operator6/1 -> Logical Operator/3
  Routine_Status/1 -> Logical Operator6/1

== system AEMS_Standard_Library/DCM/AEMS_DCM_STOP_ROUTINE/Xxx_Stop_Callback ==
  note: NRC24
  note: CLIENT/SERVER:
      |
      | ERRORCODE: Routine isn"t running ErrorCode = 36 (NRC24)
      | else ErrorCode = 0
      |
      |
      | Routine STOP Control Response:
      | Routine Status = 1 (disabled)
      | Routine Type = 3 for Renault
      | Two these values are stored in one byte dataOut_1 in which 4 LSB are for
      | Routine Status and 4 MSB are for Routine Type
      | Example: Routine Status = 1 (disabled)
      | Routine Type = 3 for Renault
      | dataOut_1: Routine Status + 2^4*Routine Type (2^4 shift 4 bits)
      | dataOut_1: 1+3*16=49
  note: routine isn"t running ErrorCode = 36 (NRC24)
      | else ErrorCode = 0
  note: CONDITION:
      |
      | case 1 : permission = 1 and previous request = 0 (init = 0)
      | 	x = permission AND NOT(previous request) = 1
      | 	y = NOT(permission) AND previous request = 1
      | 	x OR y = 1 so request = 1
      |
      | case 2 : Permission = 1 and previous request = 1
      | 	x = permission AND NOT(previous request) = 0
      | 	y = NOT(permission) AND previous request = 0
      | 	x OR y = 0 so request = 0
      |
      | case 3 : permission = 0 and previous request = 0
      | 	x = permission AND NOT(previous request) = 0
      | 	y = NOT(permission) AND previous request = 0
      | 	x OR y = 1 so request = 0
      |
      | case 4 : permission = 0 and previous request = 1
      | 	x = permission AND NOT(previous request) = 1
      | 	y = NOT(permission) AND previous request = 1
      | 	x OR y = 1 so request = 1
  note: Routine Status disable
  note: Shift Routine Type 4 bits
  note: Routine_xxxx_Status_Running
  note: E_NOT_OK
  note: E_OK
  note: Do nothing for argument OpStatus
  Routine_xxxx_Status : Inport
  OpStatus : Inport  Port=2
  Add : Sum  OutDataTypeStr=uint8  SaturateOnIntegerOverflow=on  InputSameDT=on
      settings: AttributesFormatString=SAT = %<SaturateOnIntegerOverflow>
  Constant1 : Constant  Value=0  OutDataTypeStr=uint8
  Constant2 : Constant  Value=Routine_Type_xxxx
  Constant3 : Constant  Description=NRC22  Value=0  OutDataTypeStr=uint8  SampleTime=-1
  Constant4 : Constant  Value=0  OutDataTypeStr=uint8
  ErrorCode1 : Terminator
  Logical Operator2 : Logic  OutDataTypeStr=boolean
  Logical Operator3 : Logic  Operator=NOT  OutDataTypeStr=boolean
  Logical Operator4 : Logic  OutDataTypeStr=boolean
  Logical Operator5 : Logic  Operator=NOT  OutDataTypeStr=boolean
  Logical Operator6 : Logic  Operator=OR  OutDataTypeStr=boolean
  NRC1 : Constant  Description=NRC22  OutDataTypeStr=uint8  SampleTime=-1
  NRC24 : Constant  Value=36  OutDataTypeStr=uint8
  Product : Product  OutDataTypeStr=Inherit: Inherit via back propagation  SaturateOnIntegerOverflow=on
      settings: AttributesFormatString=SAT = %<SaturateOnIntegerOverflow>
  Relational Operator : RelationalOperator  Operator===  OutDataTypeStr=boolean  RndMeth=Nearest  InputSameDT=on
  Relational Operator1 : RelationalOperator  Operator=>  OutDataTypeStr=boolean  RndMeth=Nearest  InputSameDT=on
  Routine_Status_disable : Constant  Value=Routine_Status_Aborted
  Routine_xxxx_Status_Running : Constant  Value=Routine_Status_Running
  Shift3bits : Constant  Value=16  OutDataTypeStr=uint8
  Switch : Switch  Criteria=u2 ~= 0
      settings: AttributesFormatString=Criteria=%<Criteria>
  Switch3 : Switch  Criteria=u2 ~= 0
      settings: AttributesFormatString=Criteria=%<Criteria>
  Unit Delay1 : UnitDelay  SampleTime=-1
      settings: AttributesFormatString=<initial=%<InitialCondition>>
  Flag_request_XXXX_DCM_Stop : Outport  InitialOutput=0
  dataOut_1 : Outport  Port=2  InitialOutput=0
  ErrorCode : Outport  Port=3  InitialOutput=0
  Std_ReturnType : Outport  Port=4
  wires:
  Logical Operator6/1 -> Unit Delay1/1, Flag_request_XXXX_DCM_Stop/1
  Logical Operator2/1 -> Logical Operator6/1
  Logical Operator4/1 -> Logical Operator6/2
  Logical Operator5/1 -> Logical Operator4/1
  Unit Delay1/1 -> Logical Operator3/1, Logical Operator4/2
  Logical Operator3/1 -> Logical Operator2/2
  Routine_Status_disable/1 -> Add/1
  Add/1 -> dataOut_1/1  "dataOut_1"
  Product/1 -> Add/2
  Shift3bits/1 -> Product/2
  Routine_xxxx_Status_Running/1 -> Relational Operator/2
  Switch/1 -> Relational Operator1/1, ErrorCode/1  "ErrorCode"
  NRC24/1 -> Switch/3
  Constant1/1 -> Switch/1
  Routine_xxxx_Status/1 -> Relational Operator/1
  Constant2/1 -> Product/1
  Relational Operator/1 -> Logical Operator2/1, Logical Operator5/1, Switch/2
  Switch3/1 -> Std_ReturnType/1  "Std_ReturnType"
  NRC1/1 -> Switch3/1
  Constant3/1 -> Switch3/3
  Relational Operator1/1 -> Switch3/2
  Constant4/1 -> Relational Operator1/2
  OpStatus/1 -> ErrorCode1/1

== system AEMS_Standard_Library/DEM/AEMS_DEM_SET_IUMPR_DCOND/Dem_SetIUMPRDenCondition_Call ==
  condition_status : Inport
  set_flag : EnablePort
      settings: AttributesFormatString=<states=%<StatesWhenEnabling>>
  AEMS_DEM_SETIUMPRDENCONDITION : AEMS_Standard_Library/SUB/AEMS_DEM_SETIUMPRDENCONDITION  Tag=[LIB]
      settings: AttributesFormatString=%<MaskType>
  ConditionId_Block : Constant  Value=DEM_IUMPR_GENERAL_DENOMINATOR  OutDataTypeStr=uint8
  wires:
  condition_status/1 -> AEMS_DEM_SETIUMPRDENCONDITION/2
  ConditionId_Block/1 -> AEMS_DEM_SETIUMPRDENCONDITION/1

== system AEMS_Standard_Library/DEM/AEMS_DEM_SET_OPCYC_STE/Dem_SetOperationCycleState_Call ==
  cycle_state : Inport
  call : EnablePort
      settings: AttributesFormatString=<states=%<StatesWhenEnabling>>
  AEMS_DEM_SETOPERATIONCYCLESTATE : AEMS_Standard_Library/SUB/AEMS_DEM_SETOPERATIONCYCLESTATE
      settings: AttributesFormatString=%<MaskType>
  OperationCycleId_Block : Constant  Value=DEM_OPCYC_IGNITION  OutDataTypeStr=uint8
  wires:
  OperationCycleId_Block/1 -> AEMS_DEM_SETOPERATIONCYCLESTATE/1
  cycle_state/1 -> AEMS_DEM_SETOPERATIONCYCLESTATE/2

== system AEMS_Standard_Library/DEM/AEMS_DEM_SET_PFC_CYC_QUALD/Dem_SetPfcCycleQualified_Call ==
  set_flag : EnablePort
      settings: AttributesFormatString=<states=%<StatesWhenEnabling>>
  AEMS_DEM_SETPFCCYCLEQUALIFIED : AEMS_Standard_Library/SUB/AEMS_DEM_SETPFCCYCLEQUALIFIED
      settings: AttributesFormatString=%<MaskType>

== system AEMS_Standard_Library/DISCONTINUITIES/AEMS_MULTI_PORT_TIME_SWITCH/in_clc ==
  Vsx_swi_nr : Inport  Tag=AM,In,0,1,Name,C;CMP,Port,PortWidth,SampleTime;
  Vbx_sel_puls : Inport  Tag=AM,In,0,1,Name,C;CMP,Port,PortWidth,SampleTime;  Port=2
  Vsx_sel_old : Inport  Tag=AM,In,0,1,Name,C;CMP,Port,PortWidth,SampleTime;  Port=3
  Vsx_sel : Inport  Tag=AM,In,0,1,Name,C;CMP,Port,PortWidth,SampleTime;  Port=4
  Vxx_in1 : Inport  Tag=AM,In,0,1,Name,C;CMP,Port,PortWidth,SampleTime;  Port=5
  Vxx_in2 : Inport  Tag=AM,In,0,1,Name,C;CMP,Port,PortWidth,SampleTime;  Port=6
  Vxx_in3 : Inport  Tag=AM,In,0,1,Name,C;CMP,Port,PortWidth,SampleTime;  Port=7
  Vxx_in4 : Inport  Tag=AM,In,0,1,Name,C;CMP,Port,PortWidth,SampleTime;  Port=8
  Vxx_in5 : Inport  Tag=AM,In,0,1,Name,C;CMP,Port,PortWidth,SampleTime;  Port=9
  Vxx_in6 : Inport  Tag=AM,In,0,1,Name,C;CMP,Port,PortWidth,SampleTime;  Port=10
  Vxx_in7 : Inport  Tag=AM,In,0,1,Name,C;CMP,Port,PortWidth,SampleTime;  Port=11
  Vxx_in8 : Inport  Tag=AM,In,0,1,Name,C;CMP,Port,PortWidth,SampleTime;  Port=12
  Constant1 : Constant  Tag=AM,Constant,0,1,Value;CMP,Value;  Value=2  OutDataTypeStr=Inherit: Inherit via back propagation
  Constant3 : Constant  Tag=AM,Constant,0,1,Value;CMP,Value;  OutDataTypeStr=Inherit: Inherit via back propagation
  Multiport_Switch1 : MultiPortSwitch  Tag=AM,Switch,Inputs,1;CMP,Inputs;  Inputs=8  RndMeth=Zero  SaturateOnIntegerOverflow=on  InputSameDT=on
      settings: AttributesFormatString=PortOrder=%<DataPortOrder>
  Multiport_Switch2 : MultiPortSwitch  Tag=AM,Switch,Inputs,1;CMP,Inputs;  Inputs=8  RndMeth=Zero  SaturateOnIntegerOverflow=on  InputSameDT=on
      settings: AttributesFormatString=PortOrder=%<DataPortOrder>
  Relational_Operator11 : RelationalOperator  Tag=AM,Std,2,1;CMP,Operator;  Operator===  OutDataTypeStr=boolean  RndMeth=Nearest  InputSameDT=on
  Relational_Operator41 : RelationalOperator  Tag=AM,Std,2,1;CMP,Operator;  Operator===  OutDataTypeStr=boolean  RndMeth=Nearest  InputSameDT=on
  Switch : Switch  Tag=GEN,Threshold;AM,Switch,2,1;CMP,Threshold;  Criteria=u2 ~= 0  RndMeth=Zero  SaturateOnIntegerOverflow=on  InputSameDT=on
      settings: AttributesFormatString=Criteria=%<Criteria>
  Switch1 : Switch  Tag=GEN,Threshold;AM,Switch,2,1;CMP,Threshold;  Criteria=u2 ~= 0  RndMeth=Zero  SaturateOnIntegerOverflow=on  InputSameDT=on
      settings: AttributesFormatString=Criteria=%<Criteria>
  Switch2 : Switch  Tag=GEN,Threshold;AM,Switch,2,1;CMP,Threshold;  Criteria=u2 ~= 0  RndMeth=Zero  SaturateOnIntegerOverflow=on  InputSameDT=on
      settings: AttributesFormatString=Criteria=%<Criteria>
  Unit_Delay11 : UnitDelay  Tag=GEN,X0,SampleTime;AM,Std,1,1;CMP,X0,SampleTime;  SampleTime=-1
      settings: AttributesFormatString=IC = %<X0>
  Unit_Delay3 : UnitDelay  Tag=GEN,X0,SampleTime;AM,Std,1,1;CMP,X0,SampleTime;  SampleTime=-1
      settings: AttributesFormatString=IC = %<X0>
  Vxx_out_sel : Outport  Tag=AM,Out,1,0,Name,NC;CMP,Port,OutputWhenDisabled,InitialOutput;
  Vxx_out_sel_old : Outport  Tag=AM,Out,1,0,Name,NC;CMP,Port,OutputWhenDisabled,InitialOutput;  Port=2
  wires:
  Vxx_in8/1 -> Multiport_Switch2/9, Multiport_Switch1/9
  Vxx_in7/1 -> Multiport_Switch2/8, Multiport_Switch1/8
  Vxx_in6/1 -> Multiport_Switch2/7, Multiport_Switch1/7
  Vxx_in5/1 -> Multiport_Switch2/6, Multiport_Switch1/6
  Vxx_in4/1 -> Multiport_Switch2/5, Multiport_Switch1/5
  Vxx_in3/1 -> Multiport_Switch2/4, Multiport_Switch1/4
  Vxx_in2/1 -> Multiport_Switch2/3, Multiport_Switch1/3
  Vxx_in1/1 -> Multiport_Switch2/2, Multiport_Switch1/2
  Vbx_sel_puls/1 -> Switch1/2
  Relational_Operator11/1 -> Switch2/2
  Constant1/1 -> Relational_Operator11/2
  Relational_Operator41/1 -> Switch/2
  Constant3/1 -> Relational_Operator41/2
  Multiport_Switch1/1 -> Switch2/1
  Unit_Delay11/1 -> Switch2/3
  Switch2/1 -> Unit_Delay11/1, Switch1/3
  Switch1/1 -> Vxx_out_sel_old/1
  Multiport_Switch2/1 -> Switch/1
  Unit_Delay3/1 -> Switch1/1, Switch/3
  Switch/1 -> Vxx_out_sel/1, Unit_Delay3/1
  Vsx_swi_nr/1 -> Relational_Operator41/1, Relational_Operator11/1
  Vsx_sel_old/1 -> Multiport_Switch1/1
  Vsx_sel/1 -> Multiport_Switch2/1

== system AEMS_Standard_Library/DISCONTINUITIES/AEMS_MULTI_PORT_TIME_SWITCH/interpolation ==
  Vxx_swi_trs : Inport  Tag=AM,In,0,1,Name,C;CMP,Port,PortWidth,SampleTime;
  Vbx_slop_on : Inport  Tag=AM,In,0,1,Name,C;CMP,Port,PortWidth,SampleTime;  Port=2
  Vxx_out_sel : Inport  Tag=AM,In,0,1,Name,C;CMP,Port,PortWidth,SampleTime;  Port=3
  Vxx_out_sel_old : Inport  Tag=AM,In,0,1,Name,C;CMP,Port,PortWidth,SampleTime;  Port=4
  Constant11 : Constant  Tag=AM,Constant,0,1,Value;CMP,Value;  OutDataTypeStr=Inherit: Inherit via back propagation
  Product1 : Product  Tag=AM,Std,Inputs,1;CMP,Inputs;  Inputs=**  OutDataTypeStr=Inherit: Inherit via back propagation  RndMeth=Zero
  Product2 : Product  Tag=AM,Std,Inputs,1;CMP,Inputs;  Inputs=**  OutDataTypeStr=Inherit: Inherit via back propagation  RndMeth=Zero
  Sum2 : Sum  Tag=AM,Std,Inputs,1;CMP,Inputs;  Inputs=+-  OutDataTypeStr=Inherit: Inherit via back propagation  RndMeth=Zero  InputSameDT=on
  Sum5 : Sum  Tag=AM,Std,Inputs,1;CMP,Inputs;  OutDataTypeStr=Inherit: Inherit via back propagation  RndMeth=Zero  InputSameDT=on
  Switch : Switch  Tag=GEN,Threshold;AM,Switch,2,1;CMP,Threshold;  Criteria=u2 ~= 0  RndMeth=Zero  SaturateOnIntegerOverflow=on  InputSameDT=on
      settings: AttributesFormatString=Criteria=%<Criteria>
  Vxx_out : Outport  Tag=AM,Out,1,0,Name,NC;CMP,Port,OutputWhenDisabled,InitialOutput;
  wires:
  Vxx_swi_trs/1 -> Sum2/2, Product1/1
  Vxx_out_sel/1 -> Product1/2, Switch/3
  Vxx_out_sel_old/1 -> Product2/2
  Product1/1 -> Sum5/2
  Constant11/1 -> Sum2/1
  Switch/1 -> Vxx_out/1
  Vbx_slop_on/1 -> Switch/2
  Product2/1 -> Sum5/1
  Sum5/1 -> Switch/1
  Sum2/1 -> Product2/1

== system AEMS_Standard_Library/DISCONTINUITIES/AEMS_MULTI_PORT_TIME_SWITCH/number_1_2 ==
  Vbx_slop_on : Inport  Tag=AM,In,0,1,Name,C;CMP,Port,PortWidth,SampleTime;
  Vbx_sel_puls : Inport  Tag=AM,In,0,1,Name,C;CMP,Port,PortWidth,SampleTime;  Port=2
  Constant1 : Constant  Tag=AM,Constant,0,1,Value;CMP,Value;  OutDataTypeStr=uint8
  Constant11 : Constant  Tag=AM,Constant,0,1,Value;CMP,Value;  OutDataTypeStr=Inherit: Inherit via back propagation
  Constant2 : Constant  Tag=AM,Constant,0,1,Value;CMP,Value;  Value=2  OutDataTypeStr=Inherit: Inherit via back propagation
  Logical_Operator : Logic  Tag=AM,Std,Inputs,1;CMP,Operator,Inputs;  Operator=OR  OutDataTypeStr=boolean
  Logical_Operator1 : Logic  Tag=AM,Std,Inputs,1;CMP,Operator,Inputs;  OutDataTypeStr=boolean
  Logical_Operator2 : Logic  Tag=AM,Std,Inputs,1;CMP,Operator,Inputs;  Operator=NOT  Inputs=1  OutDataTypeStr=boolean
  Relational_Operator : RelationalOperator  Tag=AM,Std,2,1;CMP,Operator;  OutDataTypeStr=boolean  RndMeth=Nearest  InputSameDT=on
  Sum2 : Sum  Tag=AM,Std,Inputs,1;CMP,Inputs;  OutDataTypeStr=Inherit: Inherit via back propagation  RndMeth=Zero  SaturateOnIntegerOverflow=on  InputSameDT=on
      settings: AttributesFormatString=SAT = %<SaturateOnIntegerOverflow>
  Switch : Switch  Tag=GEN,Threshold;AM,Switch,2,1;CMP,Threshold;  Criteria=u2 ~= 0  RndMeth=Zero  SaturateOnIntegerOverflow=on  InputSameDT=on
      settings: AttributesFormatString=Criteria=%<Criteria>
  Unit_Delay2 : UnitDelay  Tag=GEN,X0,SampleTime;AM,Std,1,1;CMP,X0,SampleTime;  InitialCondition=1  SampleTime=-1
      settings: AttributesFormatString=IC = %<X0>
  Vsx_swi_nr : Outport  Tag=AM,Out,1,0,Name,NC;CMP,Port,OutputWhenDisabled,InitialOutput;
  wires:
  Logical_Operator/1 -> Logical_Operator2/1
  Logical_Operator2/1 -> Logical_Operator1/1
  Constant2/1 -> Relational_Operator/2
  Relational_Operator/1 -> Logical_Operator/1
  Constant1/1 -> Switch/3
  Sum2/1 -> Switch/1
  Unit_Delay2/1 -> Relational_Operator/1, Sum2/1
  Constant11/1 -> Sum2/2
  Switch/1 -> Unit_Delay2/1, Vsx_swi_nr/1
  Logical_Operator1/1 -> Switch/2
  Vbx_sel_puls/1 -> Logical_Operator/2
  Vbx_slop_on/1 -> Logical_Operator1/2
